simulink model "Landing"  (R2016a)
settings: Solver=FixedStepAuto  StartTime=0.0  StopTime=120.0  FixedStep=0.1  RelTol=1e-3
libraries: simulink x1
settings Model: Creator=jason  LastModifiedBy=jason
settings SolverCC: ZeroCrossAlgorithm=Adaptive
settings GRTTargetCC: GeneratePreprocessorConditionals=Use local settings

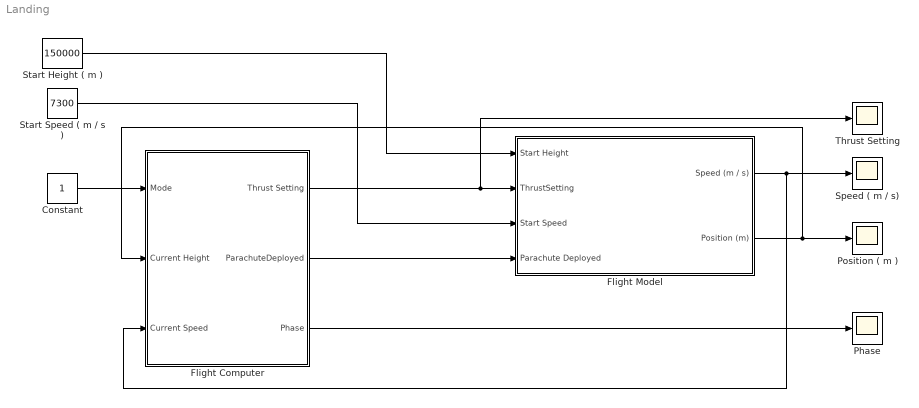
== system Landing ==
  Constant : Constant
  Flight Computer : Subsystem
  Flight Model : Subsystem  TreatAsAtomicUnit=on
      settings: MinAlgLoopOccurrences=on
  Phase : Scope
  Position ( m ) : Scope
  Speed ( m / s) : Scope
  Start Height ( m ) : Constant  Value=150000
  Start Speed ( m / s ) : Constant  Value=7300
  Thrust Setting : Scope
  wires:
  Flight Model/1(Speed (m / s)) -> Flight Computer/3(Current Speed), Speed ( m / s)/1
  Flight Model/2(Position (m)) -> Flight Computer/2(Current Height), Position ( m )/1
  Start Speed ( m / s )/1 -> Flight Model/3(Start Speed)
  Start Height ( m )/1 -> Flight Model/1(Start Height)
  Flight Computer/1(Thrust Setting) -> Thrust Setting/1, Flight Model/2(ThrustSetting)
  Constant/1 -> Flight Computer/1(Mode)
  Flight Computer/2(ParachuteDeployed) -> Flight Model/4(Parachute Deployed)
  Flight Computer/3(Phase) -> Phase/1

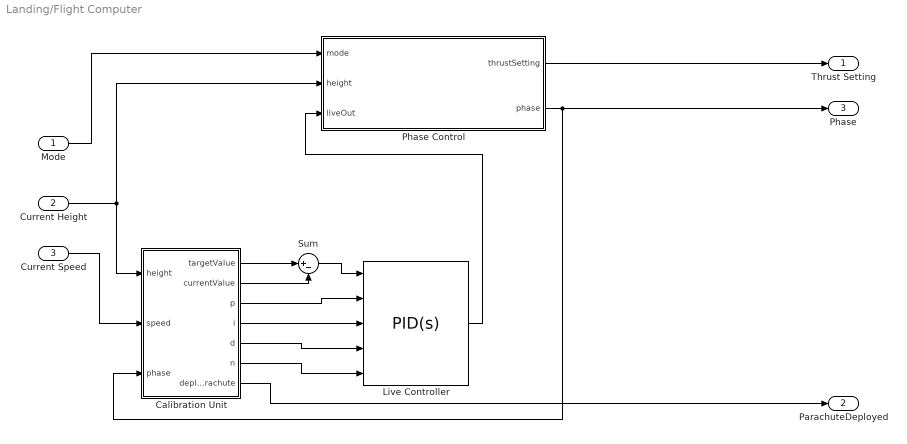
== system Landing/Flight Computer ==
  Mode : Inport
  Current Height : Inport  Port=2
  Current Speed : Inport  Port=3
  Calibration Unit : MATLAB Function  TreatAsAtomicUnit=on
  Live Controller : simulink/Continuous/PID Controller  Controller=PID  TimeDomain=Continuous-time  SampleTime=-1  IntegratorMethod=Forward Euler  FilterMethod=Forward Euler  Form=Parallel  UseFilter=on  ControllerParametersSource=external  P=1.32827832723259  I=0.287295030023929  D=0.974512189960466  N=10  InitialConditionSource=internal  InitialConditionForIntegrator=0  InitialConditionForFilter=0  ExternalReset=none  LimitOutput=on  UpperSaturationLimit=1.0  LowerSaturationLimit=0.0  LinearizeAsGain=off  AntiWindupMode=back-calculation  Kb=1  TrackingMode=off  Kt=1  PParamMin=[]  PParamMax=[]  IParamMin=[]  IParamMax=[]  DParamMin=[]  DParamMax=[]  NParamMin=[]  NParamMax=[]  KbParamMin=[]  KbParamMax=[]  KtParamMin=[]  KtParamMax=[]  POutMin=[]  POutMax=[]  IOutMin=[]  IOutMax=[]  DOutMin=[]  DOutMax=[]  NOutMin=[]  NOutMax=[]  KbOutMin=[]  KbOutMax=[]  KtOutMin=[]  KtOutMax=[]  IntegratorOutMin=[]  IntegratorOutMax=[]  FilterOutMin=[]  FilterOutMax=[]  SumOutMin=[]  SumOutMax=[]  SumI1OutMin=[]  SumI1OutMax=[]  SumI2OutMin=[]  SumI2OutMax=[]  SumI3OutMin=[]  SumI3OutMax=[]  SumDOutMin=[]  SumDOutMax=[]  SaturationOutMin=[]  SaturationOutMax=[]  IntegratorContinuousStateAttributes=''  IntegratorStateMustResolveToSignalObject=off  IntegratorRTWStateStorageClass=Auto  FilterContinuousStateAttributes=''  FilterStateMustResolveToSignalObject=off  FilterRTWStateStorageClass=Auto  DifferentiatorICPrevScaledInput=0  DifferentiatorOutMin=[]  DifferentiatorOutMax=[]
  Phase Control : MATLAB Function  TreatAsAtomicUnit=on
  Sum : Sum  Inputs=|+-
  Thrust Setting : Outport
  ParachuteDeployed : Outport  Port=2
  Phase : Outport  Port=3
  wires:
  Live Controller/1 -> Phase Control/3(liveOut)
  Mode/1 -> Phase Control/1(mode)
  Sum/1 -> Live Controller/1
  Calibration Unit/6(n) -> Live Controller/5
  Calibration Unit/5(d) -> Live Controller/4
  Calibration Unit/4(i) -> Live Controller/3
  Calibration Unit/3(p) -> Live Controller/2
  Phase Control/1(thrustSetting) -> Thrust Setting/1
  Calibration Unit/1(targetValue) -> Sum/1
  Calibration Unit/2(currentValue) -> Sum/2
  Current Height/1 -> Phase Control/2(height), Calibration Unit/1(height)
  Current Speed/1 -> Calibration Unit/2(speed)
  Phase Control/2(phase) -> Phase/1, Calibration Unit/3(phase)
  Calibration Unit/7(deployParachute) -> ParachuteDeployed/1

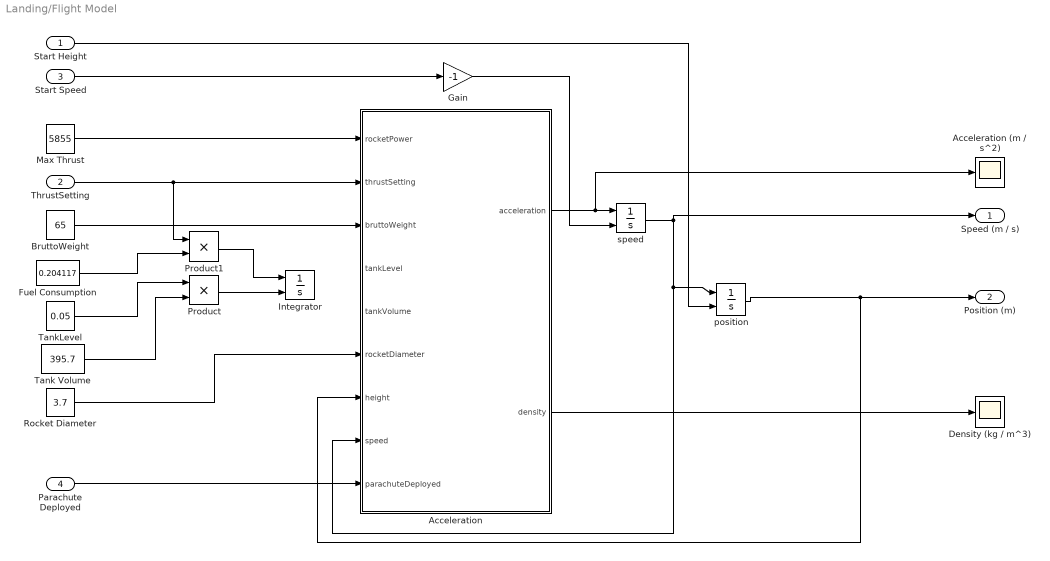
== system Landing/Flight Model ==
  Start Height : Inport
  ThrustSetting : Inport  Port=2
  Start Speed : Inport  Port=3
  Parachute Deployed : Inport  Port=4
  Acceleration : MATLAB Function  TreatAsAtomicUnit=on
  Acceleration (m / s^2) : Scope
  BruttoWeight : Constant  Value=65
  Density (kg / m^3) : Scope
  Fuel Consumption : Constant  Value=0.204117
  Gain : Gain  Gain=-1
  Integrator : Integrator  InitialConditionSource=external
  Max Thrust : Constant  Value=5855
  Product : Product
  Product1 : Product
  Rocket Diameter : Constant  Value=3.7
  Tank Volume : Constant  Value=395.7
  TankLevel : Constant  Value=0.05
  position : Integrator  InitialConditionSource=external  InitialCondition=150000
  speed : Integrator  InitialConditionSource=external
  Speed (m / s) : Outport
  Position (m) : Outport  Port=2
  wires:
  speed/1 -> Speed (m / s)/1, Acceleration/8(speed), position/1
  Rocket Diameter/1 -> Acceleration/6(rocketDiameter)
  position/1 -> Position (m)/1, Acceleration/7(height)
  Acceleration/1(acceleration) -> Acceleration (m / s^2)/1, speed/1
  Max Thrust/1 -> Acceleration/1(rocketPower)
  BruttoWeight/1 -> Acceleration/3(bruttoWeight)
  TankLevel/1 -> Product/1
  Tank Volume/1 -> Product/2
  Acceleration/2(density) -> Density (kg / m^3)/1
  ThrustSetting/1 -> Product1/1, Acceleration/2(thrustSetting)
  Gain/1 -> speed/2
  Parachute Deployed/1 -> Acceleration/9(parachuteDeployed)
  Start Speed/1 -> Gain/1
  Product/1 -> Integrator/2
  Fuel Consumption/1 -> Product1/2
  Product1/1 -> Integrator/1
  Start Height/1 -> position/2

== matlab function Landing/Flight Computer/Calibration Unit ==
  data: height input; speed input; targetValue output; currentValue output; phase input; p output; i output; d output; n output; deployParachute output
function [targetValue, currentValue, p, i, d, n, deployParachute] = calibrate(height, speed, phase)
    % Responsible for calibrating the controller's values according to
    % the current landing phase.
    
    switch phase  
            
        case 1
            targetValue = -500;
            currentValue = speed;
            p = 0.769190398299711;
            i = 1.51281865873419;
            d = -0.0284204405653449;
            n = 27.0646894628946;
            deployParachute = false;
            
        case 2
            targetValue = 0;
            currentValue = 0;
            p = 0;
            i = 0;
            d = 0;
            n = 0;
            deployParachute = true;
            
        case 3
            targetValue = -75;
            currentValue = speed;
            p = 1.32827832723259;
            i = 0.287295030023929;
            d = 0.974512189960466;
            n = 10;
            deployParachute = false;
            
        case 4
            targetValue = 0;
            currentValue = height;
            p = 1.32827832723259;
            i = 0.287295030023929;
            d = 0.974512189960466;
            n = 10;
            deployParachute = false;
            
        otherwise
            targetValue = 0;
            currentValue = 0;
            p = 0;
            i = 0;
            d = 0;
            n = 0;
            deployParachute = false;
    end

== matlab function Landing/Flight Model/Acceleration ==
  data: rocketPower input; thrustSetting input; bruttoWeight input; tankLevel input; tankVolume input; rocketDiameter input; height input; acceleration output; speed input; density output; parachuteDeployed input
function [acceleration, density ] = Acceleration( rocketPower, thrustSetting, bruttoWeight, tankLevel, tankVolume, rocketDiameter, height, speed, parachuteDeployed )
    mass = Mass(bruttoWeight, tankLevel, tankVolume);

    thrust = Thrust(thrustSetting, rocketPower, mass);
    gravity = Gravity();
    [airDrag, density] = AirDrag(speed, rocketDiameter, mass, height, parachuteDeployed);
    
    acceleration = thrust - gravity + airDrag;
end

== matlab function Landing/Flight Computer/Phase Control ==
  data: thrustSetting output; mode input; height input; phase output; liveOut input
function [thrustSetting, phase] = phaseControl(mode, height, liveOut)
    
	% Allows to switch the operating mode (if on). In "live mode", the current
	% landing phase is determined according to speed. Also, all phases can
	% be triggered directly (for experimentation and calibration purposes).
    
    % available modes    
    deactivate = 0;
    live = 1;
    expermient1 = 11;
    expermient2 = 12;
    expermient3 = 13;
    expermient4 = 14;
        
    if mode == live
        phase = determinePhase(height);        
        thrustSetting = liveOut;
    elseif mode >= expermient1 && mode <= expermient4
        phase = mode - 10;
        thrustSetting = liveOut;
    else
        thrustSetting = 0.0;
        phase = deactivate;
    end
end
    
function phase = determinePhase(height)
    
    if height <= 100
        phase = 4;        
    elseif height <= 2000
        phase = 3;
    elseif height <= 150000
        phase = 2;
    else
        phase = 0;
    end
    
end
